simulink model "Augmented"  (R2013a)
settings: Solver=ode45  StartTime=0.0  StopTime=10.0  RelTol=1e-3
settings Model: Creator=G.force  LastModifiedBy=G.force

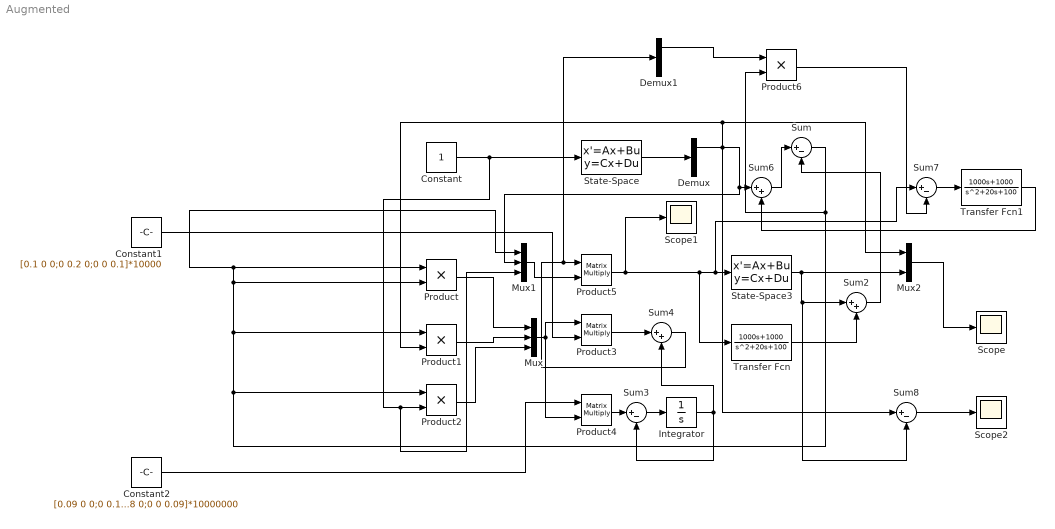
== system Augmented ==
  Constant : Constant
  Constant1 : Constant  Value=[0.1 0 0;0 0.2 0;0 0 0.1]*10000
  Constant2 : Constant  Value=[0.09 0 0;0 0.18 0;0 0 0.09]*10000000
  Demux : Demux  Outputs=2
  Demux1 : Demux  Outputs=3
  Integrator : Integrator  InitialCondition=[0.01 0.020841 1e-6]
  Mux : Mux  Inputs=3
  Mux1 : Mux  Inputs=3
  Mux2 : Mux  Inputs=2
  Product{,1..2,6} (4 alike) : Product
  Product3 : Product  Multiplication=Matrix(*)
  Product4 : Product  Multiplication=Matrix(*)
  Product5 : Product  Multiplication=Matrix(*)
  Scope : Scope
      settings: ShowLegends=on  TimeRange=4  YMin=-40  YMax=45  SaveName=sd  MaxDataPoints=100000000
  Scope1 : Scope
      settings: TimeRange=10  YMin=-4.5  YMax=4.5  SaveName=Up  MaxDataPoints=100000000
  Scope2 : Scope
      settings: ShowLegends=on  TimeRange=4  YMin=-40  YMax=45  SaveName=E  MaxDataPoints=10000000
  State-Space : StateSpace  A=[-1 0;0 -1]  B=[1;1]  C=eye(2)  D=[0;0]  X0=[0.0 0]
  State-Space3 : StateSpace  A=[0 1;-2084.1 0]  B=[0;0.9999]*1e5  C=[1 0]  D=0
  Sum{,3,7..8} (4 alike) : Sum  Inputs=|+-
  Sum2 : Sum  Inputs=|++
  Sum4 : Sum  Inputs=|++
  Sum6 : Sum  Inputs=|++
  Transfer Fcn : TransferFcn  Numerator=[1000 1000]  Denominator=[1 20 100]
  Transfer Fcn1 : TransferFcn  Numerator=[1000 1000]  Denominator=[1 20 100]
  wires:
  Constant/1 -> Mux1/3, Product2/2, State-Space/1
  Sum/1 -> Product6/2, Product2/1, Product1/1, Product/2, Product/1, Mux1/1
  Product/1 -> Mux/1
  Product1/1 -> Mux/2
  Product2/1 -> Mux/3
  Mux/1 -> Product3/1, Product4/2
  Constant1/1 -> Product3/2
  Constant2/1 -> Product4/1
  Product4/1 -> Sum3/1
  Sum3/1 -> Integrator/1
  Product3/1 -> Sum4/1
  Sum4/1 -> Demux1/1, Product5/1
  Mux1/1 -> Product5/2
  Mux2/1 -> Scope/1
  State-Space3/1 -> Sum8/2, Sum2/1, Mux2/2
  Product5/1 -> Scope1/1, Transfer Fcn/1, Sum7/1, State-Space3/1
  State-Space/1 -> Demux/1
  Transfer Fcn/1 -> Sum2/2
  Sum2/1 -> Sum/2
  Demux/1 -> Sum8/1, Product1/2, Mux2/1, Mux1/2, Sum6/1
  Transfer Fcn1/1 -> Sum6/2
  Sum6/1 -> Sum/1
  Demux1/1 -> Product6/1
  Sum7/1 -> Transfer Fcn1/1
  Product6/1 -> Sum7/2
  Sum8/1 -> Scope2/1
  Integrator/1 -> Sum3/2, Sum4/2
